simulink model "pidtestmodel"  (R2023b)
settings: Solver=VariableStepAuto  StartTime=0.0  StopTime=100.0  RelTol=1e-3
settings Model: Creator=12183  LastModifiedBy=12183

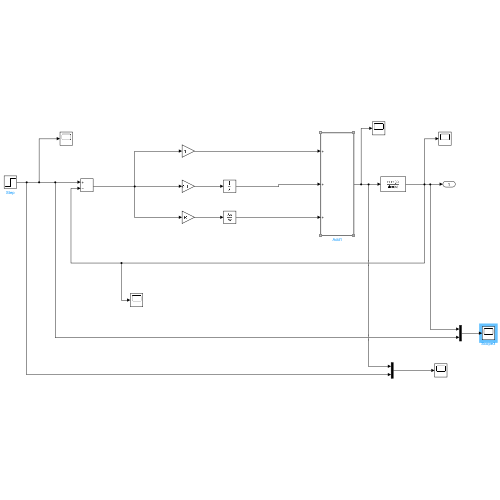
[thumbnail: Simulink's stored preview of the top-level diagram]
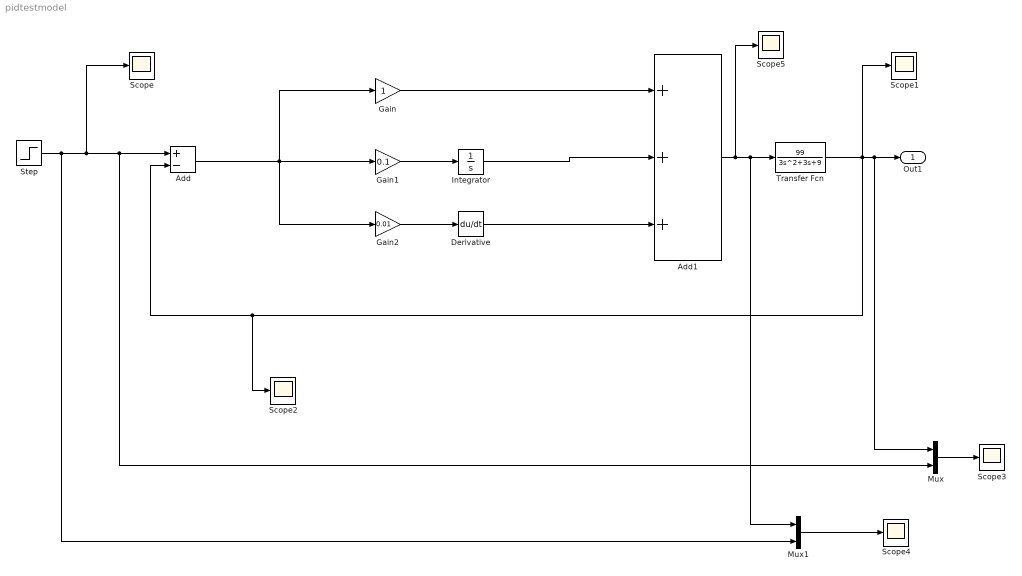
== system pidtestmodel ==
  Add : Sum  Inputs=+-
  Add1 : Sum  Inputs=+++
  Derivative : Derivative
  Gain : Gain
  Gain1 : Gain  Gain=0.1
  Gain2 : Gain  Gain=0.01
  Integrator : Integrator
  Mux : Mux  Inputs=2
  Mux1 : Mux  Inputs=2
  Scope{,1..5} (6 alike) : Scope
  Step : Step  SampleTime=0
  Transfer Fcn : TransferFcn  Numerator=[99]  Denominator=[3 3 9]
  Out1 : Outport
  wires:
  Gain1/1 -> Integrator/1
  Gain2/1 -> Derivative/1
  Integrator/1 -> Add1/2
  Add/1 -> Gain2/1, Gain/1, Gain1/1
  Gain/1 -> Add1/1
  Derivative/1 -> Add1/3
  Step/1 -> Mux1/2, Scope/1, Mux/2, Add/1
  Add1/1 -> Scope5/1, Mux1/1, Transfer Fcn/1
  Transfer Fcn/1 -> Scope2/1, Add/2, Scope1/1, Mux/1, Out1/1
  Mux/1 -> Scope3/1
  Mux1/1 -> Scope4/1
